simulink model "epex9Diagram"  (R2021a)
settings: Solver=FixedStepAuto  StartTime=0.0  StopTime=100  FixedStep=0.5  RelTol=1e-3
undefined symbols (not defined in the file): a, am, b, bm, R1, S0, S1
settings Model: Creator=dbnun  LastModifiedBy=dbnun

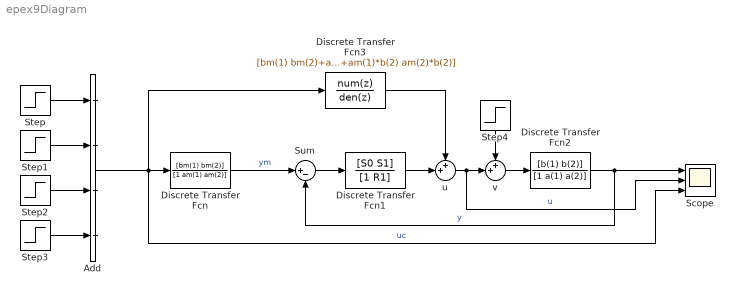
== system epex9Diagram ==
  Add : Sum  Inputs=++++
  Discrete Transfer Fcn : DiscreteTransferFcn  Numerator=[bm(1) bm(2)]  Denominator=[1 am(1) am(2)]  SampleTime=0.5
  Discrete Transfer Fcn1 : DiscreteTransferFcn  Numerator=[S0 S1]  Denominator=[1 R1]
  Discrete Transfer Fcn2 : DiscreteTransferFcn  Numerator=[b(1) b(2)]  Denominator=[1 a(1) a(2)]
  Discrete Transfer Fcn3 : DiscreteTransferFcn  Numerator=[bm(1) bm(2)+a(1)*bm(1) a(1)*bm(2)+a(2)*bm(1) a(2)*bm(2)]  Denominator=[b(1) b(2)+b(1)*am(1) am(2)*b(1)+am(1)*b(2) am(2)*b(2)]
  Scope : Scope  NumInputPorts=3
  Step : Step  Time=0  SampleTime=0
  Step1 : Step  Time=25  After=-2  SampleTime=0
  Step2 : Step  Time=50  After=2  SampleTime=0
  Step3 : Step  Time=75  After=-2  SampleTime=0
  Step4 : Step  Time=40  After=0.5  SampleTime=0
  Sum : Sum  Inputs=|+-
  u : Sum  Inputs=++|
  v : Sum  Inputs=++|
  wires:
  Step2/1 -> Add/3
  Step1/1 -> Add/2
  Add/1 -> Scope/3, Discrete Transfer Fcn3/1, Discrete Transfer Fcn/1  "uc"
  Step/1 -> Add/1
  Step3/1 -> Add/4
  Discrete Transfer Fcn/1 -> Sum/1  "ym"
  Sum/1 -> Discrete Transfer Fcn1/1
  Discrete Transfer Fcn1/1 -> u/2
  u/1 -> Scope/2, v/2  "u"
  Discrete Transfer Fcn2/1 -> Scope/1, Sum/2  "y"
  Discrete Transfer Fcn3/1 -> u/1
  v/1 -> Discrete Transfer Fcn2/1
  Step4/1 -> v/1
